simulink subsystem "DCGearmotorResonant_SubSystem"  (R2020b)
settings: Solver=VariableStepAuto  StartTime=0.0  StopTime=10.0  RelTol=1e-3
values from neighbouring files (symbols this model uses):
  rads2rpm = 60/2/pi    (= 9.54929658551)    [load_params_resonant_case.m]
settings Model: Creator=umberto  LastModifiedBy=umberto

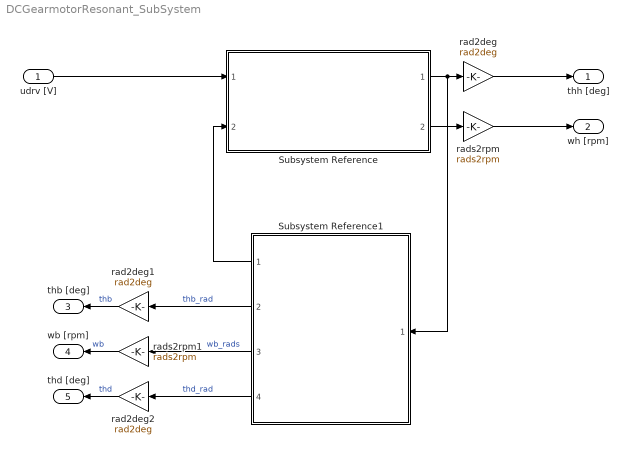
== system DCGearmotorResonant_SubSystem ==
  udrv [V] : Inport
  Subsystem Reference : Subsystem  ReferencedSubsystem=DCGearbox_SubSystem
  Subsystem Reference1 : Subsystem  ReferencedSubsystem=ResonantLoad_SubSystem
  rad2deg : Gain  Gain=rad2deg
  rad2deg1 : Gain  Gain=rad2deg
  rad2deg2 : Gain  Gain=rad2deg
  rads2rpm : Gain  Gain=rads2rpm
  rads2rpm1 : Gain  Gain=rads2rpm
  thh [deg] : Outport
  wh [rpm] : Outport  Port=2
  thb [deg] : Outport  Port=3
  wb [rpm] : Outport  Port=4
  thd [deg] : Outport  Port=5
  wires:
  udrv [V]/1 -> Subsystem Reference/1
  Subsystem Reference/1 -> Subsystem Reference1/1, rad2deg/1
  Subsystem Reference/2 -> rads2rpm/1
  rads2rpm/1 -> wh [rpm]/1
  rad2deg/1 -> thh [deg]/1
  Subsystem Reference1/1 -> Subsystem Reference/2
  Subsystem Reference1/2 -> rad2deg1/1  "thb_rad"
  Subsystem Reference1/3 -> rads2rpm1/1  "wb_rads"
  Subsystem Reference1/4 -> rad2deg2/1  "thd_rad"
  rad2deg2/1 -> thd [deg]/1  "thd"
  rads2rpm1/1 -> wb [rpm]/1  "wb"
  rad2deg1/1 -> thb [deg]/1  "thb"
